simulink model "xilinx_hw_test_au50_16k_8in"  (R2021a)
settings: Solver=VariableStepDiscrete  StartTime=0.0  StopTime=1024*2  RelTol=1e-3
undefined symbols (not defined in the file): d0, d1, d2, d3, d4, d5, d6, d7, sr
libraries: xbsIndex_r4 x1266, xrbsSSR_Library x13, casper_library_misc x7, xps_library x1
(part 2 of 18)

== system xilinx_hw_test_au50_16k_8in/bram_in0 ==
  addr : Inport
  data_in : Inport  Port=2
  we : Inport  Port=3
  Terminator : Terminator
  Terminator1 : Terminator
  Terminator2 : Terminator
  calc_add : Subsystem  mask{data_width=32, addr_width=11, sample_rate=sample_rate}
      mask prompts: data_width "data width"; addr_width "address width"; sample_rate "sample rate"
  convert_addr : xbsIndex_r4/Convert  gui_display_data_type=Fixed-point  arith_type=Unsigned  n_bits=addr_width  bin_pt=0  float_type=Single  exp_bits=8  fraction_bits=24  quantization=Truncate  overflow=Wrap  en=off  latency=0  pipeline=off  dbl_ovrd=off  block_type=convert
      settings: xl_area=[0, 0, 0, 0, 0, 0, 0]
  convert_din1 : xbsIndex_r4/Convert  gui_display_data_type=Fixed-point  arith_type=Unsigned  n_bits=32  bin_pt=0  float_type=Single  exp_bits=8  fraction_bits=24  quantization=Truncate  overflow=Wrap  en=off  latency=0  pipeline=off  dbl_ovrd=off  block_type=convert
      settings: xl_area=[0, 0, 0, 0, 0, 0, 0]
  convert_we : xbsIndex_r4/Convert  gui_display_data_type=Fixed-point  arith_type=Unsigned  n_bits=1  bin_pt=0  float_type=Single  exp_bits=8  fraction_bits=24  quantization=Truncate  overflow=Wrap  en=off  latency=0  pipeline=off  dbl_ovrd=off  block_type=convert
      settings: xl_area=[0, 0, 0, 0, 0, 0, 0]
  munge_in : Subsystem  AncestorBlock=casper_library_flow_control/munge  mask(munge){divisions=1, div_size=32, order=[0], arith_type_out=Unsigned, bin_pt_out=0}
      mask prompts: divisions "Number of divisions"; div_size "Division size (bits)"; order "Division packing order"; arith_type_out "Output arithmetic type"; bin_pt_out "Output binary point"
      mask help: Splits an input bus into the specified number of divisions and then recombines them in the order specified (most significant division = 0,least = number divisions-1)
      mask init:
      | munge_init(gcb, ...
      |     'divisions', divisions, ...
      |     'div_size', div_size, ...
      |     'order', order, ...
      |     'arith_type_out', arith_type_out, ...
      |     'bin_pt_out', bin_pt_out);
      settings: AttributesFormatString=|
      | split:32
      | join:0
      | Unsigned [32,0]
      mask TypeOptions arith_type_out: Unsigned | Signed  (2's comp) | Floating-point
  munge_out : Subsystem  AncestorBlock=casper_library_flow_control/munge  mask(munge){divisions=1, div_size=32, order=[0], arith_type_out=Signed  (2's comp), bin_pt_out=0}
      mask prompts: divisions "Number of divisions"; div_size "Division size (bits)"; order "Division packing order"; arith_type_out "Output arithmetic type"; bin_pt_out "Output binary point"
      mask help: Splits an input bus into the specified number of divisions and then recombines them in the order specified (most significant division = 0,least = number divisions-1)
      mask init:
      | munge_init(gcb, ...
      |     'divisions', divisions, ...
      |     'div_size', div_size, ...
      |     'order', order, ...
      |     'arith_type_out', arith_type_out, ...
      |     'bin_pt_out', bin_pt_out);
      settings: AttributesFormatString=|
      | split:32
      | join:0
      | Signed  (2's comp) [32,0]
      mask TypeOptions arith_type_out: Unsigned | Signed  (2's comp) | Floating-point
  sim_mem : Subsystem  mask{arith_type=Signed  (2's comp), addr_width=11, data_width=32, data_bin_pt=0, init_vals=[1955   -783   8673   3057    502  -3416   -695  -2762  -2454   1293   7946  -6381  -3299   4876   8392   1841   3917   7083   3941  -1683  -1392   5033   -637   1524  -1151   2939  -5379   7110   6719  -1947  -1047  -8591  -4813   2319     54     44  -4892   3868  -2970   1082   4131   4137  -4745   1584   1471  -4149   2972   -348   2818  -2754    293   -177   -115  -5990   1812   1094   3121   4631   -611  -6224   2980    573   7535   6280  -3513   5430  -5379   1895  -4657   -696   -392   -741  -2142   1080   2941   1562    331   -850  -3788   -495   1798   1349   1760   6351   1856   5174    691   -965  -2279   7788   -204   2427    843    379  -4266  -1542  -3474    746   3033   2338   5614   2572  -1161   3707   5579   3400   6105   1907  -3653   2239  -4023  -4168   6934  -3337   2155   6660  -1421   6722  -8797  -2565   2533  -4794   3317   1310  -5455   1455   -163 -11262   1331   2800  -9404  -1879    250   5558   6913  -7412  -1651  -1733   1994    748   5619   -493  -4417  -7232  -4489  -3772   1676  -2928  -2388    316  -2279   5744   4465    351   3456   1831  -6721   -131  -1324   4465  -1945   2137   1759  -2404  13311  -3231   2575  -5274   7490   2852   2433  -2470   -562   6461   1271   2229  -2454   -963  -1235  -2221   -884   4993  -4686   -623   2609  -1091  -1744   1350  -2187  -3974  -4542    937  -3543  -1777  12537  -3639  -8467  -1634   5494  -7915  -1426  -2424  -1244   1945   2591   1931   1325   2812   1541  -6413  -8861  -5957    778   -643  -4404  -2747  -2107  -2842   6110   9265   3664  -3103   1420  -1468  -4676   2828   4433  -1980    665  -2200  -1527   -724  -3404  -5721  -5276  -2466   4392   1731  -2439   3349  -7454   3376  -2091   4298   -127   3643   8300   -140   1289   1919  -5979    725   3320   2732   2491  -1757  -7711   6611  -6128   1712  10157   3211    782  -5771   3862  -7351  -6269   9702  -1503  -2901   3900    999  -6646   4870   3523  -1996  -3592   6041  -2440    446  -4550  -5848  -5127  -5769  -3026   2337   -377   3280   -361  -3151   1474   2780  -3106  -5715  -1194  -8906   2933   5649  -3955  -3475  -3851   -161    913   2318   7838  -2884   1930  -6759   4374   -105  -3750    452  -4449   -635   -600  -6927   3731  -4213  -4289  -1327   4870  -1732   7211   7961   2070   -179  -3374    -57  -3526   5108   5523   1280  -2744   4166  -3007  -4720  -3246  -3541  -4326   1494  -2077   2525    872  -2608  -2298  -1990   1883   3096    209  -5760   5269   2514   1840   4112  -6776  -1005   1052  -1369  -3480   1898   2121   5096    569  -1512    969   4956   5318     93 -12520   2354  -2261  -2039  -1936  -4223   1084  -8327   1722  -2927  -1785    102   -499  -6808   1059    909  -6021   1054   3844   -961   2879  -4608    474  -8316  -2505  -5706  -2435   1650   2510  -5770  -1159   -177   4224   2927   5845   1448    207    145    557    251   3689   1293   -492     18  -2611  13891   3951  -5884  -2674  -3366   3851    537   4585   5700   1327  -5332  -4464  -2075  -3855  -1703   -261 -10904  -3609   4305   6782  -1758   3020     -4  -3207    326   6219   1986   4399   1282   -195  -5283  -1907  -2272  -1780   6557  -1132   8083  -1397   1890  -9297   3287   1206  -3967  -5320  -7897  -9623    557  -3415   3125  -1248   -387   2140   -859   4286   4530   -741   4036   3123   6359  -2092   1657   -327  -6391   1297    618   3480    102   2532  11033    460   5688   4963  -4496  -4280    265   1266    850   1633  -3111   -296  -2746   -623   1250  -4330   1440  -5660   -103   5739  -5331   2836   2365  -4297  -4697   1340  -3338  -2008    493    918  -3354  -7002  -7336  -6296   1464  -2154    999  -8681   -523  -2554  -3734    329  -5662   2966   2895   6828  -8507  -1016   -689  -1945   1455   3223   2011  -1146  -1052  -3857  -3211   2405  -3924  -1048  -4623  -1137  -5341   -728  -5684    636   1305   1554   1207   9185  -3090   1511  -3454    931   -692  -2158  -1392   9433    -45   -151  -4418   -822   2971   9750  -3463  -4669    533   4846   6378  -6282 ...(+10338 chars)], sample_rate=1, csp_latency=1}
      mask prompts: arith_type "Output Data Type"; addr_width "Address width"; data_width "Data width"; data_bin_pt "Data Binary Point"; init_vals "Initial values"; sample_rate "Sample rate"; csp_latency "Latency"
      mask init:
      | % set_param([gcb, '/data_to_xilinx'], 'arith_type', arith_type)
      | % set_param([gcb, '/data_to_xilinx'], 'n_bits', get_param(gcb, 'data_width'))
      mask TypeOptions arith_type: Unsigned | Signed  (2's comp)
      mask TypeOptions data_width: 8 | 16 | 32 | 64 | 128
  xilinx_hw_test_au50_16k_8in_bram_in0_addr : xbsIndex_r4/Gateway Out  inherit_from_input=off  hdl_port=on  rows=1  columns=1  UseAsDAC=off  DACChannel='1'  interface=None  automatic_assignment=on  address_offset=hex2dec('00')  intf_name=''  intf_description=''  timing_constraint=None  locs_specified=off  LOCs={'A5','B9','A9','C1','A3','G6','E9','A6','A7','A8','B8','B1','B3','D9','B5','B4','B6','C2'}  io_standard={}  block_type=gatewayout
      settings: infoedit="Gateway out block.  Converts Xilinx fixed point inputs into ouputs of type Simulink integer, double, or fixed point.<P><P>Hardware notes:  In hardware these blocks become top level output ports or are discarded, depending on how they are configured."  sginterface={'Nallatech'=>{'xdspkit'=>{'non_memory_mapped_port'=>'uprev_Shared_BRAM_addr'}},'Xilinx'=>{'jtaghwcosim'=>{'non_memory_mapped_port'=>'uprev_Shared_BRAM_addr'},'xdspkit'=>{'non_memory_mapped_port'=>'uprev_Shared_BRAM_addr'}}}  xl_area=[0, 0, 0, 0, 0, 0, 0]
  xilinx_hw_test_au50_16k_8in_bram_in0_data_in : xbsIndex_r4/Gateway Out  inherit_from_input=off  hdl_port=on  rows=1  columns=1  UseAsDAC=off  DACChannel='1'  interface=None  automatic_assignment=on  address_offset=hex2dec('00')  intf_name=''  intf_description=''  timing_constraint=None  locs_specified=off  LOCs={'B21','B22','A22','B23','B19','C19','A20','A21','A23','B24','A24','A25','E18','D18','C18','B18'}  io_standard={}  block_type=gatewayout
      settings: infoedit="Gateway out block.  Converts Xilinx fixed point inputs into ouputs of type Simulink integer, double, or fixed point.<P><P>Hardware notes:  In hardware these blocks become top level output ports or are discarded, depending on how they are configured."  sginterface={'Nallatech'=>{'xdspkit'=>{'non_memory_mapped_port'=>'uprev_Shared_BRAM_data_in'}},'Xilinx'=>{'jtaghwcosim'=>{'non_memory_mapped_port'=>'uprev_Shared_BRAM_data_in'},'xdspkit'=>{'non_memory_mapped_port'=>'uprev_Shared_BRAM_data_in'}}}  xl_area=[0, 0, 0, 0, 0, 0, 0]
  xilinx_hw_test_au50_16k_8in_bram_in0_data_out : xbsIndex_r4/Gateway In  gui_display_data_type=Fixed-point  arith_type=Unsigned  n_bits=32  bin_pt=0  preci_type=Single  exp_width=8  frac_width=24  rows=1  columns=1  quantization=Truncate  overflow=Wrap  period=sample_rate  UseAsADC=off  ADCChannel='1'  interface=None  automatic_assignment=on  address_offset=hex2dec('00')  intf_name=''  intf_description=''  default_value=0  timing_constraint=None  locs_specified=off  LOCs={}  io_standard={}  inherit_from_input=off  hdl_port=on  dbl_ovrd=off  block_type=gatewayin
      settings: xl_area=[0, 0, 0, 0, 0, 0, 0]
  xilinx_hw_test_au50_16k_8in_bram_in0_we : xbsIndex_r4/Gateway Out  inherit_from_input=off  hdl_port=on  rows=1  columns=1  UseAsDAC=off  DACChannel='1'  interface=None  automatic_assignment=on  address_offset=hex2dec('00')  intf_name=''  intf_description=''  timing_constraint=None  locs_specified=off  LOCs={'A14'}  io_standard={}  block_type=gatewayout
      settings: infoedit="Gateway out block.  Converts Xilinx fixed point inputs into ouputs of type Simulink integer, double, or fixed point.<P><P>Hardware notes:  In hardware these blocks become top level output ports or are discarded, depending on how they are configured."  xl_area=[0, 0, 0, 0, 0, 0, 0]
  data_out : Outport  VectorParamsAs1DForOutWhenUnconnected=off
  wires:
  munge_out/1(dout) -> data_out/1
  sim_mem/1(data_out) -> xilinx_hw_test_au50_16k_8in_bram_in0_data_out/1
  xilinx_hw_test_au50_16k_8in_bram_in0_data_out/1 -> munge_out/1(din)
  convert_addr/1 -> xilinx_hw_test_au50_16k_8in_bram_in0_addr/1
  convert_din1/1 -> xilinx_hw_test_au50_16k_8in_bram_in0_data_in/1
  data_in/1 -> munge_in/1(din)
  calc_add/1(out) -> convert_addr/1
  xilinx_hw_test_au50_16k_8in_bram_in0_we/1 -> Terminator2/1
  xilinx_hw_test_au50_16k_8in_bram_in0_data_in/1 -> Terminator1/1
  xilinx_hw_test_au50_16k_8in_bram_in0_addr/1 -> Terminator/1
  convert_we/1 -> xilinx_hw_test_au50_16k_8in_bram_in0_we/1
  addr/1 -> sim_mem/1(addr), calc_add/1(in)
  we/1 -> sim_mem/3(we), convert_we/1
  munge_in/1(dout) -> sim_mem/2(data), convert_din1/1

== system xilinx_hw_test_au50_16k_8in/bram_in1 ==
  addr : Inport
  data_in : Inport  Port=2
  we : Inport  Port=3
  Terminator : Terminator
  Terminator1 : Terminator
  Terminator2 : Terminator
  calc_add : Subsystem  mask{data_width=32, addr_width=11, sample_rate=sample_rate}
      mask prompts: data_width "data width"; addr_width "address width"; sample_rate "sample rate"
  convert_addr : xbsIndex_r4/Convert  gui_display_data_type=Fixed-point  arith_type=Unsigned  n_bits=addr_width  bin_pt=0  float_type=Single  exp_bits=8  fraction_bits=24  quantization=Truncate  overflow=Wrap  en=off  latency=0  pipeline=off  dbl_ovrd=off  block_type=convert
      settings: xl_area=[0, 0, 0, 0, 0, 0, 0]
  convert_din1 : xbsIndex_r4/Convert  gui_display_data_type=Fixed-point  arith_type=Unsigned  n_bits=32  bin_pt=0  float_type=Single  exp_bits=8  fraction_bits=24  quantization=Truncate  overflow=Wrap  en=off  latency=0  pipeline=off  dbl_ovrd=off  block_type=convert
      settings: xl_area=[0, 0, 0, 0, 0, 0, 0]
  convert_we : xbsIndex_r4/Convert  gui_display_data_type=Fixed-point  arith_type=Unsigned  n_bits=1  bin_pt=0  float_type=Single  exp_bits=8  fraction_bits=24  quantization=Truncate  overflow=Wrap  en=off  latency=0  pipeline=off  dbl_ovrd=off  block_type=convert
      settings: xl_area=[0, 0, 0, 0, 0, 0, 0]
  munge_in : Subsystem  AncestorBlock=casper_library_flow_control/munge  mask(munge){divisions=1, div_size=32, order=[0], arith_type_out=Unsigned, bin_pt_out=0}
      mask prompts: divisions "Number of divisions"; div_size "Division size (bits)"; order "Division packing order"; arith_type_out "Output arithmetic type"; bin_pt_out "Output binary point"
      mask help: Splits an input bus into the specified number of divisions and then recombines them in the order specified (most significant division = 0,least = number divisions-1)
      mask init:
      | munge_init(gcb, ...
      |     'divisions', divisions, ...
      |     'div_size', div_size, ...
      |     'order', order, ...
      |     'arith_type_out', arith_type_out, ...
      |     'bin_pt_out', bin_pt_out);
      settings: AttributesFormatString=|
      | split:32
      | join:0
      | Unsigned [32,0]
      mask TypeOptions arith_type_out: Unsigned | Signed  (2's comp) | Floating-point
  munge_out : Subsystem  AncestorBlock=casper_library_flow_control/munge  mask(munge){divisions=1, div_size=32, order=[0], arith_type_out=Signed  (2's comp), bin_pt_out=0}
      mask prompts: divisions "Number of divisions"; div_size "Division size (bits)"; order "Division packing order"; arith_type_out "Output arithmetic type"; bin_pt_out "Output binary point"
      mask help: Splits an input bus into the specified number of divisions and then recombines them in the order specified (most significant division = 0,least = number divisions-1)
      mask init:
      | munge_init(gcb, ...
      |     'divisions', divisions, ...
      |     'div_size', div_size, ...
      |     'order', order, ...
      |     'arith_type_out', arith_type_out, ...
      |     'bin_pt_out', bin_pt_out);
      settings: AttributesFormatString=|
      | split:32
      | join:0
      | Signed  (2's comp) [32,0]
      mask TypeOptions arith_type_out: Unsigned | Signed  (2's comp) | Floating-point
  sim_mem : Subsystem  mask{arith_type=Signed  (2's comp), addr_width=11, data_width=32, data_bin_pt=0, init_vals=[1984   5930  -1496    264 -11500   2816  -3465   4211   6657    705    302  11510  -3511  -4006    615   2073  -3380  -4164  -3764  -3852  -2893  -1352  -3318  -1048   1398    -41   2741  -3047   4740  -2802  -1780   -464   8910   2850  -5526  -3618  -2938   2713  -1390   -154  -3020  -8336    857   1784   4311    881  -1465   4417   1117   6053  -1071  -4228  -2884   -837  -1377   1408  -1868  -2380  -4225   -586  -7881   2206    444  -9734   -597  -7634   6561  -5544   -730  -6910   5936  -3620    353   1431   -714  -3555  -3170   1947  -1442   1094    123   2125  -6534   1989  10081   -798    541   3322   3350  -2357   4959   6155  -1055   4652   2781    173   8718  -5542  -3142  -1370   -961    510  -1795   -168   -469  -1197   8129  -6588   5796    598  -3096 -11313   2411  -9921   1039  -2910  -1849   4123   4656    948  -5002   7833   6143   3754   7336   5582  -1221  -5287   3237   1840   -248  -3411  -6395  -2522   -822  -4702   2657  -2382   1402   7362  -1933   5599   5292  -8979    211  -2990   7315  -1155    333   3303   9631 -13279  -7533  -4806    516   5311   -813  -9049   -640   -868  -9784   4103  -1607   1767   1847   -195  -1699  -3463  -2448  -6614   5710  -7816   5820  -1350   4878   3668  -1589   4066   -647   -130  -1059   1501   2933     67    286  -2646   6765  -1103   4745  -4242   2507  -3883   2094  -1839   2093    226   1916    497  -4396  -5275   2871   -789   2358    564  -5137  -3902  -1511    -19  -5473  -6474   6195  -6542     97  -4414   9057  -1026  -1206   4491   3214  -8910   9374  -3176   -867  -2676   -986   4379   1612  -7989  -1137  -7967     99   6480    949  -4649  -6252  -3421  -6975    434  -4961  -1437   6867   -826  -3300  -4196   2009   -968    772   -380   2307   -739  -4145   -915   3058  -2795   -819  -2081  -1469    896  -3690   4741  -2699  -1671   3480  -3929    868  -2774   1304  -3706    787    482   -735  -3180   -617  -2513   8394   -586  -4140   2696  -6628   6262  -3956   -443   6253 -11463   -285  -3345  -5511   4465   7853  -7882   4968  -6292  -1167  -4054  -3462  -7422  -8289  -3825    466   -299   2980   6431   2501  -4104  -2526  -1877   2090    627  -1640  -2780   5024   2331  -2143    562  -1945   3558  -1390  -4427    961   -986  15001   -995  -4907   3820   -193   -340    491  -1012    861  -6570  11622  -1583   5971   4553  -1249    401   4552  -5853   -847   6680   1522   -818  -7221  -3838   2128   6253  -2816  -8955     -2  -1512  -1592  -5394 -10615   1316   1577  -3231  -2196   2704  -8406  -3274   3901   8959  -6286   4389   1151  -3111   8700 -10143   1702  -7383   6299   -882  -8867   -789   1229  -2349    371  -4029    834   6094  -2253  -3192  -1614  -6930   2314    -99   6106   1854    641   4618   2084  -6271   2221   9671  -3459   7380   1993   4505   3572  -3905  -1839   4991   1879   7812    607  -5094  -1452  -6816   3910  -4306     80  -2276   5415   2353  -1264   4460   -971  -3881   -227  -5878   4650  -3723  -1772   7156   5133  -1656  -1967   3131   3156  -1984    385  -4320   4929  -3881   1134   6806   5057  -1196   2075   9722    465    614   4368    110   3823    858   -211  -9639    824    148  -2536   2970  -8633  -3342  -1964   5269   1927   1884   1213   2999  -3946  -4089   4536    916  -2996  -4168     84  -6205  -4637   1906    600   -248  -7519   4791  -1950   -989  -5421  -3022  -5703   1258  -2772   5588  -2079  -5219  -1645  -4101  -1555   -294  -3611   1635     87   -225    -64   -410   1446   1938   4065    543  -2390  -7665  -3827    884  -7881   1205  -2050   1661    178  -6949   2808  -7818    -59  -7440   -410   1336   3431  -5307   5686   1083   1545  -5735  -4192   2721   2946   1376   2572  -1312   4635  -2887    427  -1739  -1138  -5880  -2527  -3727   4563  -3622   1847  -1182   1441   2436  -5260   -565   3514  -5314  -6584   1656   3058   5330  -1299   4332   1322   5253  -4402   7598   3384    662  -4694   2887   1544   2626  -1513  -6894   -412   6067   7673    366   2241  -5750   2824  -5720  -2109 ...(+10338 chars)], sample_rate=1, csp_latency=1}
      mask prompts: arith_type "Output Data Type"; addr_width "Address width"; data_width "Data width"; data_bin_pt "Data Binary Point"; init_vals "Initial values"; sample_rate "Sample rate"; csp_latency "Latency"
      mask init:
      | % set_param([gcb, '/data_to_xilinx'], 'arith_type', arith_type)
      | % set_param([gcb, '/data_to_xilinx'], 'n_bits', get_param(gcb, 'data_width'))
      mask TypeOptions arith_type: Unsigned | Signed  (2's comp)
      mask TypeOptions data_width: 8 | 16 | 32 | 64 | 128
  xilinx_hw_test_au50_16k_8in_bram_in1_addr : xbsIndex_r4/Gateway Out  inherit_from_input=off  hdl_port=on  rows=1  columns=1  UseAsDAC=off  DACChannel='1'  interface=None  automatic_assignment=on  address_offset=hex2dec('00')  intf_name=''  intf_description=''  timing_constraint=None  locs_specified=off  LOCs={'A5','B9','A9','C1','A3','G6','E9','A6','A7','A8','B8','B1','B3','D9','B5','B4','B6','C2'}  io_standard={}  block_type=gatewayout
      settings: infoedit="Gateway out block.  Converts Xilinx fixed point inputs into ouputs of type Simulink integer, double, or fixed point.<P><P>Hardware notes:  In hardware these blocks become top level output ports or are discarded, depending on how they are configured."  sginterface={'Nallatech'=>{'xdspkit'=>{'non_memory_mapped_port'=>'uprev_Shared_BRAM_addr'}},'Xilinx'=>{'jtaghwcosim'=>{'non_memory_mapped_port'=>'uprev_Shared_BRAM_addr'},'xdspkit'=>{'non_memory_mapped_port'=>'uprev_Shared_BRAM_addr'}}}  xl_area=[0, 0, 0, 0, 0, 0, 0]
  xilinx_hw_test_au50_16k_8in_bram_in1_data_in : xbsIndex_r4/Gateway Out  inherit_from_input=off  hdl_port=on  rows=1  columns=1  UseAsDAC=off  DACChannel='1'  interface=None  automatic_assignment=on  address_offset=hex2dec('00')  intf_name=''  intf_description=''  timing_constraint=None  locs_specified=off  LOCs={'B21','B22','A22','B23','B19','C19','A20','A21','A23','B24','A24','A25','E18','D18','C18','B18'}  io_standard={}  block_type=gatewayout
      settings: infoedit="Gateway out block.  Converts Xilinx fixed point inputs into ouputs of type Simulink integer, double, or fixed point.<P><P>Hardware notes:  In hardware these blocks become top level output ports or are discarded, depending on how they are configured."  sginterface={'Nallatech'=>{'xdspkit'=>{'non_memory_mapped_port'=>'uprev_Shared_BRAM_data_in'}},'Xilinx'=>{'jtaghwcosim'=>{'non_memory_mapped_port'=>'uprev_Shared_BRAM_data_in'},'xdspkit'=>{'non_memory_mapped_port'=>'uprev_Shared_BRAM_data_in'}}}  xl_area=[0, 0, 0, 0, 0, 0, 0]
  xilinx_hw_test_au50_16k_8in_bram_in1_data_out : xbsIndex_r4/Gateway In  gui_display_data_type=Fixed-point  arith_type=Unsigned  n_bits=32  bin_pt=0  preci_type=Single  exp_width=8  frac_width=24  rows=1  columns=1  quantization=Truncate  overflow=Wrap  period=sample_rate  UseAsADC=off  ADCChannel='1'  interface=None  automatic_assignment=on  address_offset=hex2dec('00')  intf_name=''  intf_description=''  default_value=0  timing_constraint=None  locs_specified=off  LOCs={}  io_standard={}  inherit_from_input=off  hdl_port=on  dbl_ovrd=off  block_type=gatewayin
      settings: xl_area=[0, 0, 0, 0, 0, 0, 0]
  xilinx_hw_test_au50_16k_8in_bram_in1_we : xbsIndex_r4/Gateway Out  inherit_from_input=off  hdl_port=on  rows=1  columns=1  UseAsDAC=off  DACChannel='1'  interface=None  automatic_assignment=on  address_offset=hex2dec('00')  intf_name=''  intf_description=''  timing_constraint=None  locs_specified=off  LOCs={'A14'}  io_standard={}  block_type=gatewayout
      settings: infoedit="Gateway out block.  Converts Xilinx fixed point inputs into ouputs of type Simulink integer, double, or fixed point.<P><P>Hardware notes:  In hardware these blocks become top level output ports or are discarded, depending on how they are configured."  xl_area=[0, 0, 0, 0, 0, 0, 0]
  data_out : Outport  VectorParamsAs1DForOutWhenUnconnected=off
  wires:
  munge_out/1(dout) -> data_out/1
  sim_mem/1(data_out) -> xilinx_hw_test_au50_16k_8in_bram_in1_data_out/1
  xilinx_hw_test_au50_16k_8in_bram_in1_data_out/1 -> munge_out/1(din)
  convert_addr/1 -> xilinx_hw_test_au50_16k_8in_bram_in1_addr/1
  convert_din1/1 -> xilinx_hw_test_au50_16k_8in_bram_in1_data_in/1
  data_in/1 -> munge_in/1(din)
  calc_add/1(out) -> convert_addr/1
  xilinx_hw_test_au50_16k_8in_bram_in1_we/1 -> Terminator2/1
  xilinx_hw_test_au50_16k_8in_bram_in1_data_in/1 -> Terminator1/1
  xilinx_hw_test_au50_16k_8in_bram_in1_addr/1 -> Terminator/1
  convert_we/1 -> xilinx_hw_test_au50_16k_8in_bram_in1_we/1
  addr/1 -> sim_mem/1(addr), calc_add/1(in)
  we/1 -> sim_mem/3(we), convert_we/1
  munge_in/1(dout) -> sim_mem/2(data), convert_din1/1
